simulink model "rocky_motor_disturb_5_poles"  (R2021b)
settings: Solver=VariableStepAuto  StartTime=0.0  StopTime=2  RelTol=1e-3
model workspace (MAT data in the model file):
  m = 1000
values from neighbouring files (symbols this model uses):
  g = 9.81    [Rocky_closed_loop_poles.m]    (also in rocky_constants.m)
  ki = real(1.241009049348965e+05)    [rocky_constants.m]
  kp = real(1.240922125348965e+05)    [rocky_constants.m]
  l = 22*2.54/100    (= 0.5588)    [Rocky_closed_loop_poles.m]    (also in rocky_constants.m)
undefined symbols (not defined in the file or in its folder): Ci, Ji, Jp
settings Model: Creator=clee1  LastModifiedBy=spoka
settings SolverCC: AlgebraicLoopSolver=TrustRegion
settings DebuggingCC: SFMachineParentedDataDiag=warning

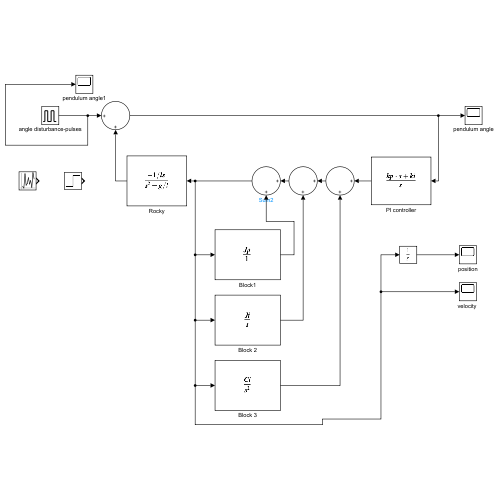
[thumbnail: Simulink's stored preview of the top-level diagram]
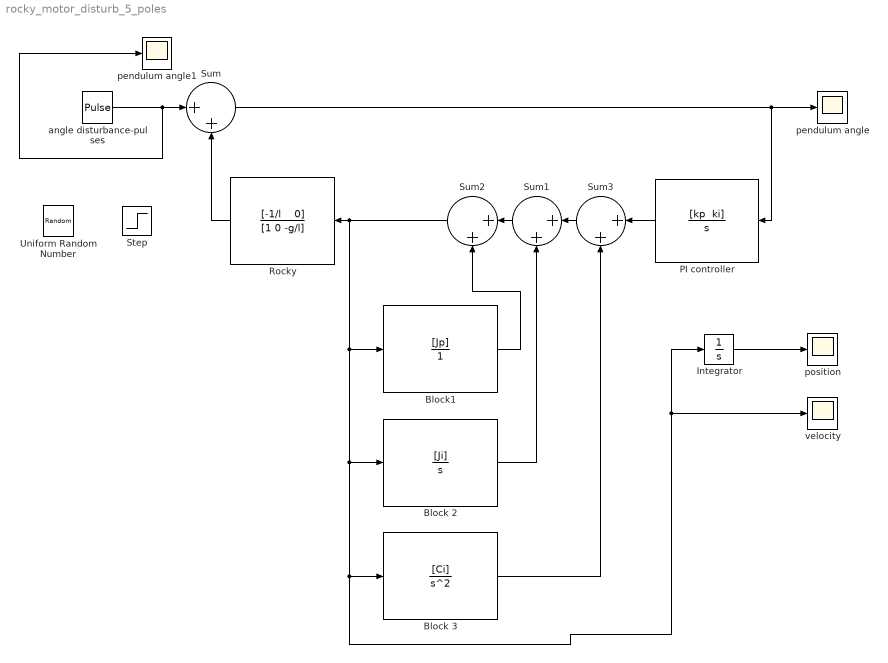
== system rocky_motor_disturb_5_poles ==
  Block 2 : TransferFcn  Numerator=[Ji]  Denominator=[1 0 ]
  Block 3 : TransferFcn  Numerator=[Ci]  Denominator=[1 0 0 ]
  Block1 : TransferFcn  Numerator=[Jp]  Denominator=[1]
  Integrator : Integrator
  PI controller : TransferFcn  Numerator="[kp  ki]"  Denominator=[1 0 ]
  Rocky : TransferFcn  Numerator="[-1/l    0]"  Denominator=[1 0 -g/l]
  Step : Step  After=.1  SampleTime=0
  Sum{,1..3} (4 alike) : Sum  Inputs=|++
  Uniform Random Number : UniformRandomNumber  SampleTime=20
  angle disturbance-pulses : DiscretePulseGenerator  PulseType=Time based  Amplitude=.1  Period=10  PulseWidth=.1  PhaseDelay=.5
  pendulum angle : Scope
  pendulum angle1 : Scope
  position : Scope
  "velocity " : Scope
  wires:
  Sum/1 -> PI controller/1, pendulum angle/1
  Integrator/1 -> position/1
  angle disturbance-pulses/1 -> pendulum angle1/1, Sum/1
  Sum1/1 -> Sum2/1
  Sum3/1 -> Sum1/1
  Block1/1 -> Sum2/2
  Block 2/1 -> Sum1/2
  Block 3/1 -> Sum3/2
  PI controller/1 -> Sum3/1
  Sum2/1 -> Block1/1, Block 2/1, Block 3/1, Integrator/1, "velocity "/1, Rocky/1
  Rocky/1 -> Sum/2
